simulink model "EOR"  (R2020b)
settings: Solver=FixedStepAuto  StartTime=0.0  StopTime=TMax  FixedStep=DT  RelTol=1e-3  EnableMultiTasking=on
values from neighbouring files (symbols this model uses):
  g = gearbox_ratio    [EOR_CSTmod_init.m]    (also in EOR_init.m = @(theta) f(v_x_breakpoints(k),theta))
  rho = 1.225    [BLCTRL_init.m]    (also in EOR_init.m)
  theta_star = interp1(v_x_breakpoints, theta_star_lookup, windspeed)    [EOR_CSTmod_init.m]
undefined symbols (not defined in the file or in its folder): C_d, CP, CP_lambda, CP_star, CP_theta, EOR_filt_a, EOR_filt_b, EOR_Omega_star_lookup, EOR_pitch_A, EOR_pitch_B, EOR_pitch_Ce, EOR_pitch_Dew, EOR_pitch_F, EOR_pitch_thresh, EOR_T, EOR_T_avg, EOR_T_solve, EOR_theta_star_lookup, EOR_torque, EOR_torque_LQR_R, EOR_v_x_breakpoints, J_g, J_r, K_d, lambda_star, Omega_rated, R
libraries: ctrlSharedLib x1
settings Model: Creator=lpwoolcock  LastModifiedBy=lpwoolcock

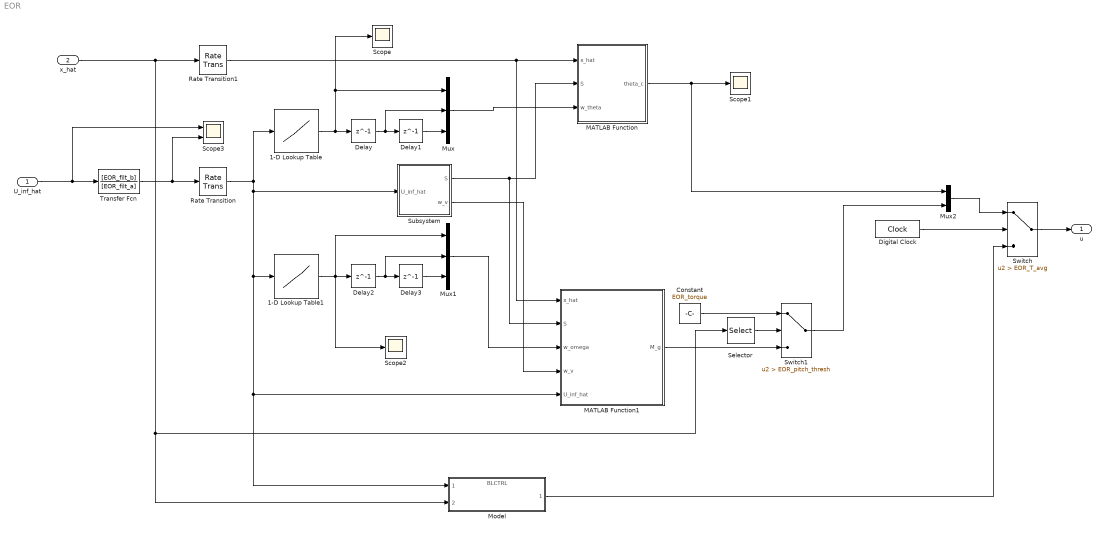
== system EOR ==
  U_inf_hat : Inport  PortDimensions=1
  x_hat : Inport  Port=2  PortDimensions=[5 1]
  1-D Lookup Table : Lookup_n-D  NumberOfTableDimensions=1  BreakpointsForDimension1=EOR_v_x_breakpoints  Table=EOR_theta_star_lookup  InternalRulePriority=Speed  RndMeth=Simplest  InputSameDT=on
  1-D Lookup Table1 : Lookup_n-D  NumberOfTableDimensions=1  BreakpointsForDimension1=EOR_v_x_breakpoints  Table=EOR_Omega_star_lookup  InternalRulePriority=Speed  RndMeth=Simplest  InputSameDT=on
  Constant : Constant  Value=EOR_torque
  Delay{,1..3} (4 alike) : Delay  DelayLength=1
  Digital Clock : DigitalClock  SampleTime=EOR_T
  MATLAB Function : MATLAB Function  TreatAsAtomicUnit=on
  MATLAB Function1 : MATLAB Function  TreatAsAtomicUnit=on
  Model : ModelReference  ModelNameDialog=BLCTRL.slx  SimulationMode=Normal  ModelReferenceVersion=2.4
  Mux : Mux  Inputs=3
  Mux1 : Mux  Inputs=3
  Mux2 : Mux  Inputs=2
  Rate Transition : RateTransition  OutPortSampleTime=EOR_T
  Rate Transition1 : RateTransition  InitialCondition=zeros(5,1)  OutPortSampleTime=EOR_T
  Scope : Scope
  Scope1 : Scope
  Scope2 : Scope
  Scope3 : Scope  NumInputPorts=2
  Selector : Selector  InputPortWidth=5  IndexOptions=Index vector (dialog)  Indices=4  OutputSizes=1
  Subsystem : Subsystem
  Switch : Switch  Criteria=u2 > Threshold  Threshold=EOR_T_avg
  Switch1 : Switch  Criteria=u2 > Threshold  Threshold=EOR_pitch_thresh
  Transfer Fcn : TransferFcn  Numerator=[EOR_filt_b]  Denominator=[EOR_filt_a]
  u : Outport  PortDimensions=[2 1]
  wires:
  Switch/1 -> u/1
  x_hat/1 -> Rate Transition1/1, Selector/1, Model/2
  Delay/1 -> Mux/2, Delay1/1
  1-D Lookup Table/1 -> Scope/1, Mux/1, Delay/1
  Delay1/1 -> Mux/3
  Delay3/1 -> Mux1/3
  Delay2/1 -> Mux1/2, Delay3/1
  1-D Lookup Table1/1 -> Scope2/1, Mux1/1, Delay2/1
  Subsystem/1(S) -> MATLAB Function1/2(S), MATLAB Function/2(S)
  Mux/1 -> MATLAB Function/3(w_theta)
  MATLAB Function/1(theta_c) -> Scope1/1, Mux2/1
  Mux2/1 -> Switch/1
  Model/1 -> Switch/3
  Digital Clock/1 -> Switch/2
  Subsystem/2(w_v) -> MATLAB Function1/4(w_v)
  Mux1/1 -> MATLAB Function1/3(w_omega)
  Rate Transition/1 -> Subsystem/1(U_inf_hat), Model/1, MATLAB Function1/5(U_inf_hat), 1-D Lookup Table1/1, 1-D Lookup Table/1
  Rate Transition1/1 -> MATLAB Function1/1(x_hat), MATLAB Function/1(x_hat)
  Transfer Fcn/1 -> Scope3/2, Rate Transition/1
  U_inf_hat/1 -> Scope3/1, Transfer Fcn/1
  MATLAB Function1/1(M_g) -> Switch1/3
  Switch1/1 -> Mux2/2
  Selector/1 -> Switch1/2
  Constant/1 -> Switch1/1

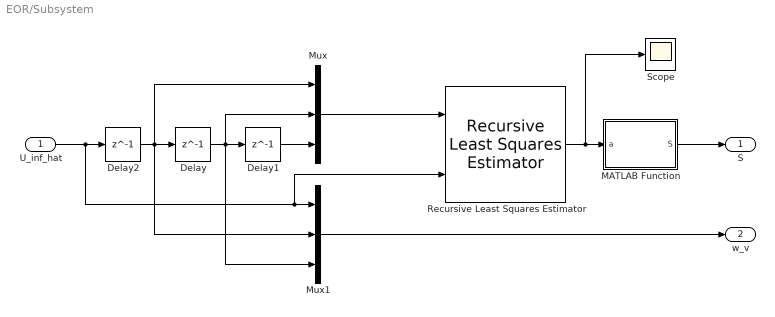
== system EOR/Subsystem ==
  U_inf_hat : Inport
  Delay : Delay  DelayLength=1
  Delay1 : Delay  DelayLength=1
  Delay2 : Delay  DelayLength=1
  MATLAB Function : MATLAB Function  TreatAsAtomicUnit=on
  Mux : Mux  Inputs=3
  Mux1 : Mux  Inputs=3
  Recursive Least Squares Estimator : ctrlSharedLib/Recursive Least Squares Estimator  InitialEstimateSource=None  InitialParameterData=3  P0=1e4  InitialRegressors=0  InitialOutputs=0  History=Infinite  WindowLength=200  EstimationMethod=Forgetting Factor  AdaptationParameter=0.99  HasTimeVaryingAdaptationParameter=off  NormalizationBias=eps  OutputError=off  OutputP=off  AddEnablePort=off  InputProcessing=Sample-based  Ts=EOR_T
      settings: SourceProductBaseCode=CT,ID
  Scope : Scope
  S : Outport
  w_v : Outport  Port=2
  wires:
  Delay/1 -> Mux1/3, Mux/2, Delay1/1
  Delay1/1 -> Mux/3
  Delay2/1 -> Mux1/2, Mux/1, Delay/1
  U_inf_hat/1 -> Recursive Least Squares Estimator/2, Mux1/1, Delay2/1
  Mux/1 -> Recursive Least Squares Estimator/1
  Mux1/1 -> w_v/1
  Recursive Least Squares Estimator/1 -> Scope/1, MATLAB Function/1(a)
  MATLAB Function/1(S) -> S/1

== matlab function EOR/MATLAB Function ==
  data: x_hat input size=[5 1]; theta_c output; S input size=[3 3]; w_theta input; EOR_pitch_A parameter size=[2 2]; EOR_pitch_B parameter size=[2 1]; EOR_pitch_Ce parameter size=[1 2]; EOR_pitch_Dew parameter size=[1 3]; EOR_pitch_F parameter size=[1 2]; EOR_T_avg parameter size=1; EOR_T parameter size=1; EOR_T_solve parameter size=1
function theta_c = EOR_pitch(x_hat, S, w_theta, EOR_pitch_A, EOR_pitch_B, EOR_pitch_Ce, EOR_pitch_Dew, EOR_pitch_F, EOR_T_avg, EOR_T, EOR_T_solve)

    persistent t;
    if isempty(t)
        t = 0;
    end
    
    persistent G;

    if t < EOR_T_avg && isempty(G)
        theta_c = 0;
    else
        if isempty(G) || t > EOR_T_solve
            
            Gamma = zeros(1, 3);
            Pi = zeros(2, 3);
            [Pi, Gamma] = EOR_solve(EOR_pitch_A, EOR_pitch_B, zeros(2, 3),...
                EOR_pitch_Ce, 0, EOR_pitch_Dew, S);
            G = Gamma - EOR_pitch_F * Pi;
            
            t = 0;
        end
        
        theta_c = EOR_pitch_F*x_hat(4:5) + G*w_theta;
    end
    
    
    t = t + EOR_T;
end

== matlab function EOR/Subsystem/MATLAB Function ==
  data: a input; S output size=[3 3]
function S = fcn(a)

    S = [a(1) a(2) a(3); 1 0 0; 0 1 0];

end

== matlab function EOR/MATLAB Function1 ==
  data: x_hat input size=[5 1]; M_g output; S input size=[3 3]; w_omega input; w_v input size=[3 1]; U_inf_hat input; EOR_T_avg parameter size=1; EOR_T parameter size=1; EOR_T_solve parameter size=1; EOR_torque_LQR_R parameter; Omega_rated parameter; R parameter size=1; rho parameter size=1; CP parameter; CP_lambda parameter; CP_theta parameter; C_d parameter size=1; J_r parameter size=1; K_d parameter size=1; g parameter size=1; J_g parameter size=1; CP_star parameter size=1; theta_star parameter size=1; lambda_star parameter size=1
function M_g = EOR_torque(x_hat, S, w_omega, w_v, U_inf_hat, EOR_T_avg, EOR_T, EOR_T_solve, EOR_torque_LQR_R, Omega_rated, R, rho, CP, CP_lambda, CP_theta, C_d, J_r, K_d, g, J_g, CP_star, theta_star, lambda_star)

    persistent t vx0;
    if isempty(t)
        t = 0;
        vx0 = 0;
    end
    
    persistent F G;
    
    persistent A B Ew Ce Dew;
    persistent x_star u_star;
    
    coder.extrinsic('dlqr');
    
    if t < EOR_T_avg && isempty(G)
        M_g = 0;
        
        vx0 = vx0 + U_inf_hat * EOR_T / EOR_T_avg;
    else
        if isempty(G)
            % calculate equilibrium point and produce linearised system
            % matrices

            
            vx0 = min(vx0, Omega_rated * R / lambda_star);
            
            u_star = 0.5e-6 * rho * pi * R^3 * CP_star / lambda_star * vx0^2; % in MNm
            Omega_r_star = lambda_star * vx0 / R;
            x_star = [Omega_r_star; u_star/(1e-9*K_d); Omega_r_star];
            
            [theta_grid, lambda_grid] = meshgrid(CP_theta, CP_lambda);
            lambda = @(Omega_r, vx) Omega_r * R / vx;
            M_a = @(Omega_r, vx, theta) 0.5 * rho * pi * R^3 * vx^2 ...
                * interp2(theta_grid, lambda_grid, CP, theta, lambda(Omega_r, vx), 'cubic') ...
                / lambda(Omega_r, vx);

            d_vx = 0.001;
            alpha = (M_a(Omega_r_star, vx0 + d_vx, theta_star)...
                - M_a(Omega_r_star, vx0, theta_star)) / d_vx;

            d_Omega_r = 0.001;
            gamma = (M_a(Omega_r_star + d_Omega_r, vx0, theta_star)...
                - M_a(Omega_r_star, vx0, theta_star)) / d_Omega_r;
    
            A_c = [(gamma - C_d)/J_r -K_d/(1000*J_r) C_d/J_r; 1000 0 -1000;...
                    C_d/(g*J_g) K_d/(1000*g*J_g) -C_d/(g*J_g)];
            B_c = [0;
                   0;
                  -1e6/(g*J_g)];
            Ew_c = [alpha/J_r zeros(1,5);zeros(2,6)];

            A = expm(A_c*EOR_T);
            B = A_c\(A-eye(size(A)))*B_c;
            Ce = [1 0 0];
            Ew = A_c\(A-eye(size(A)))*Ew_c;
            Dew = [0 0 0 -1 0 0];
            
            K = zeros(1,3);
            [K, ~, ~] = dlqr(A, B, 1, EOR_torque_LQR_R);
            F = -K;
            G = zeros(1,6);
        end
        
        if t > EOR_T_solve
            Gamma = zeros(1, 6);
            Pi = zeros(3, 6);
            
            S_T = [S zeros(3); zeros(3) S];
            
            [Pi, Gamma] = EOR_solve(A, B, Ew, Ce, 0, Dew, S_T);
            G = Gamma - F * Pi;
            
            t = 0;
        end
        
        M_g = F*(x_hat(1:3) - x_star) + G*[(w_v - vx0); (w_omega - x_star(1))] + u_star;
    end
    
    
    t = t + EOR_T;
end
